simulink model "LKA_Lenkung_CarMaker_DSR_kombiniert_algSynth"  (Simulink 7.9)
settings: Solver=ode23  StartTime=0.0  StopTime=tend-1  FixedStep=0.01  RelTol=1e-3
undefined symbols (not defined in the file or in its folder): pin
libraries: library x5, simulink x3
settings Model: Creator=Georg  LastModifiedBy=georgnestlinger
settings DebuggingCC: FcnCallInpInsideContextMsg=Use local settings  StrictBusMsg=Warning
settings GRTTargetCC: CombineOutputUpdateFcns=off  GRTInterface=on

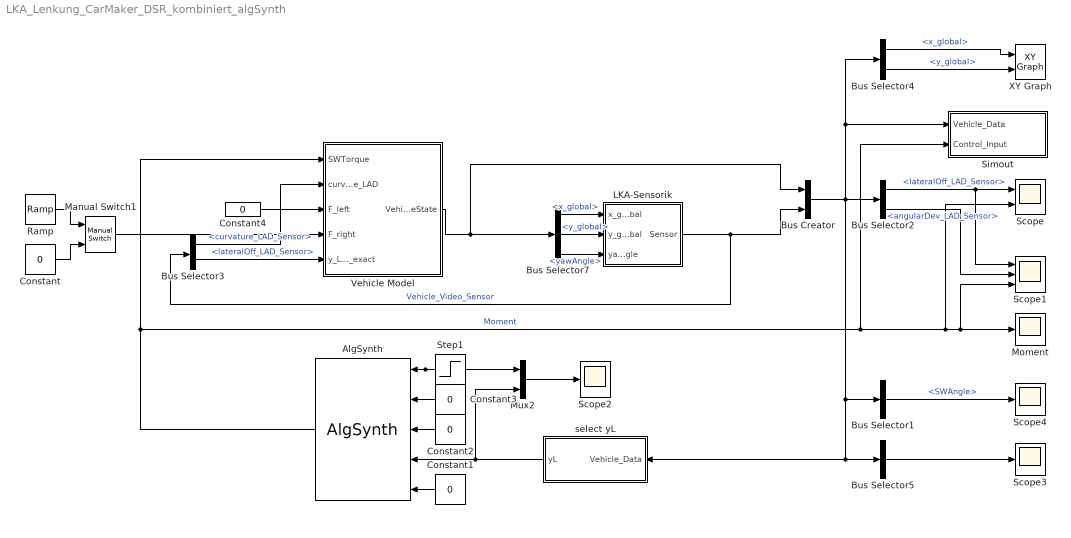
== system LKA_Lenkung_CarMaker_DSR_kombiniert_algSynth ==
  AlgSynth : library/LKA-Controller/AlgSynth
  Bus Creator : BusCreator  Inputs=2
  Bus Selector1 : BusSelector  OutputSignals=VehicleState.SWAngle
  Bus Selector2 : BusSelector  OutputSignals=Vehicle_Video_Sensor.lateralOff_LAD_Sensor,Vehicle_Video_Sensor.angularDev_LAD_Sensor
  Bus Selector3 : BusSelector  OutputSignals=curvature_LAD_Sensor,lateralOff_LAD_Sensor
  Bus Selector4 : BusSelector  OutputSignals=VehicleState.x_global,VehicleState.y_global
  Bus Selector5 : BusSelector  OutputSignals=VehicleState.angularDev_LAD_nonlinear,Vehicle_Video_Sensor.angularDev_LAD_Sensor  OutputAsBus=on
  Bus Selector7 : BusSelector  OutputSignals=x_global,y_global,yawAngle
  Constant{,1..4} (5 alike) : Constant  Value=0
  LKA-Sensorik : Subsystem  BlockChoice=Videosensorik
      settings: AttributesFormatString=%<BlockChoice>  TemplateBlock=library/LKA-Sensorik/LKA-Sensorik  MemberBlocks=Videosensorik
  Manual Switch1 : simulink/Signal Routing/Manual Switch  sw=0  action=0  varsize=off
  Moment : Scope
      settings: TimeRange=32.2  YMin=0.0002694  YMax=0.0002697  SaveName=ScopeData2
  Mux2 : Mux  Inputs=2
  Ramp : simulink/Sources/Ramp  slope=1  start=20  X0=0
  Scope : Scope  NumInputPorts=2
      settings: TimeRange=12.7664  YMin=-2.5e-06~-5e-05  YMax=3.25e-05~0.00025
  Scope1 : Scope  NumInputPorts=3
      settings: TimeRange=20  YMin=-5.5e-008~0.01711~-1.666e-008  YMax=5e-009~0.017145~-1.6565e-008
  Scope2 : Scope
      settings: TimeRange=5.66  YMin=0  YMax=1.05e-008  SaveName=ScopeData6
  Scope3 : Scope
      settings: YMin=0  YMax=0.035  SaveName=ScopeData3
  Scope4 : Scope
      settings: YMin=0.1675  YMax=0.205  SaveName=ScopeData4
  Simout : Subsystem
  Step1 : Step  Time=10  After=0  SampleTime=0
  Vehicle Model : Subsystem
  XY Graph : simulink/Sinks/XY Graph  xmin=-100  xmax=700  ymin=-1  ymax=600  st=-1
  select yL : Subsystem  BlockChoice=yL_Sensor
      settings: AttributesFormatString=%<BlockChoice>  TemplateBlock=library/LKA-Sensorik/select yL  MemberBlocks=yL_Sensor,yL_exactMdl,yL_linMdl
  wires:
  Bus Selector4/1 -> XY Graph/1  "<x_global>"
  Bus Selector4/2 -> XY Graph/2  "<y_global>"
  Bus Selector2/1 -> Scope/1, Scope1/1  "<lateralOff_LAD_Sensor>"
  Bus Selector2/2 -> Scope1/2  "<angularDev_LAD_Sensor>"
  Vehicle Model/1(VehicleState) -> Bus Creator/1, Bus Selector7/1
  LKA-Sensorik/1(Sensor) -> Bus Creator/2, Bus Selector3/1  "Vehicle_Video_Sensor"
  Bus Creator/1 -> Bus Selector2/1, Bus Selector1/1, Bus Selector5/1, select yL/1(Vehicle_Data), Bus Selector4/1, Simout/1(Vehicle_Data)
  Bus Selector5/1 -> Scope3/1
  Bus Selector1/1 -> Scope4/1  "<SWAngle>"
  Constant/1 -> Manual Switch1/2
  Manual Switch1/1 -> Vehicle Model/4(F_right)
  Bus Selector3/2 -> Vehicle Model/5(y_LAD_exact)  "<lateralOff_LAD_Sensor>"
  Bus Selector3/1 -> Vehicle Model/2(curvature_LAD)  "<curvature_LAD_Sensor>"
  select yL/1(yL) -> Mux2/2, AlgSynth/4
  AlgSynth/1 -> Scope/2, Scope1/3, Moment/1, Simout/2(Control_Input), Vehicle Model/1(SWTorque)  "Moment"
  Mux2/1 -> Scope2/1
  Step1/1 -> Mux2/1, AlgSynth/1
  Constant3/1 -> AlgSynth/2
  Constant2/1 -> AlgSynth/3
  Constant1/1 -> AlgSynth/5
  Constant4/1 -> Vehicle Model/3(F_left)
  Ramp/1 -> Manual Switch1/1
  Bus Selector7/1 -> LKA-Sensorik/1(x_global)  "<x_global>"
  Bus Selector7/2 -> LKA-Sensorik/2(y_global)  "<y_global>"
  Bus Selector7/3 -> LKA-Sensorik/3(yawAngle)  "<yawAngle>"

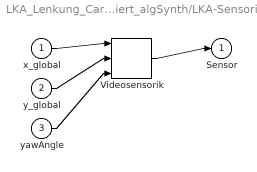
== system LKA_Lenkung_CarMaker_DSR_kombiniert_algSynth/LKA-Sensorik ==
  x_global : Inport
  y_global : Inport  Port=2
  yawAngle : Inport  Port=3
  Videosensorik : library/LKA-Sensorik/Videosensorik
  Sensor : Outport
  wires:
  x_global/1 -> Videosensorik/1
  y_global/1 -> Videosensorik/2
  yawAngle/1 -> Videosensorik/3
  Videosensorik/1 -> Sensor/1

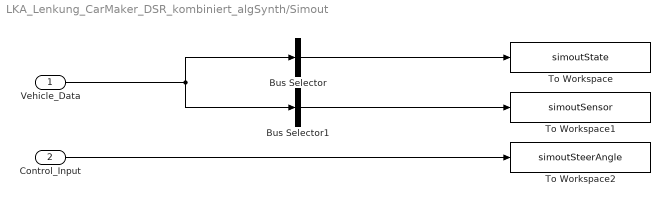
== system LKA_Lenkung_CarMaker_DSR_kombiniert_algSynth/Simout ==
  Vehicle_Data : Inport
  Control_Input : Inport  Port=2
  Bus Selector : BusSelector  OutputSignals=VehicleState  OutputAsBus=on
  Bus Selector1 : BusSelector  OutputSignals=Vehicle_Video_Sensor  OutputAsBus=on
  To Workspace : ToWorkspace  VariableName=simoutState  SampleTime=-1  SaveFormat=Structure With Time
  To Workspace1 : ToWorkspace  VariableName=simoutSensor  SampleTime=-1  SaveFormat=Structure With Time
  To Workspace2 : ToWorkspace  VariableName=simoutSteerAngle  SampleTime=-1  SaveFormat=Structure With Time
  wires:
  Vehicle_Data/1 -> Bus Selector1/1, Bus Selector/1
  Control_Input/1 -> To Workspace2/1
  Bus Selector/1 -> To Workspace/1
  Bus Selector1/1 -> To Workspace1/1

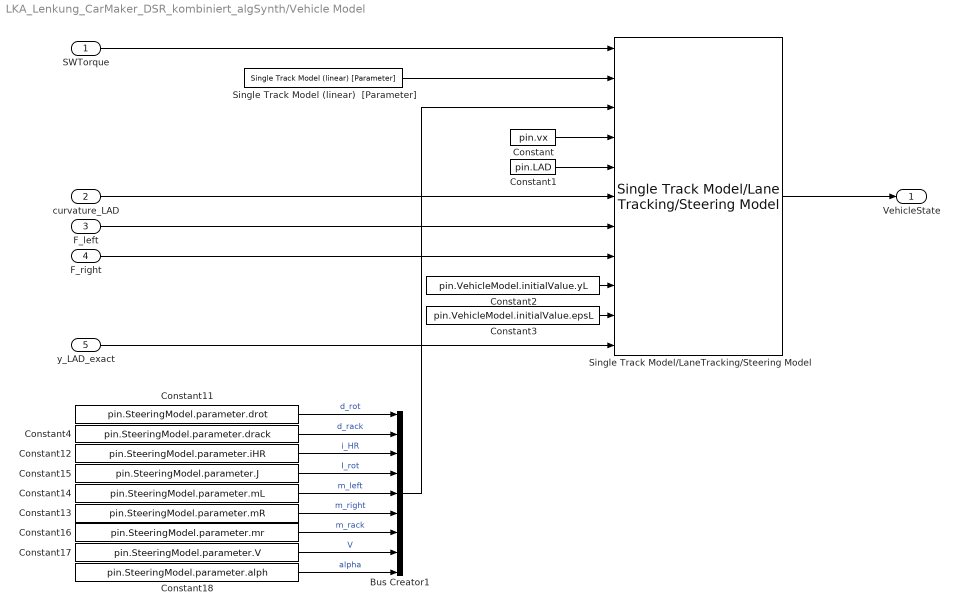
== system LKA_Lenkung_CarMaker_DSR_kombiniert_algSynth/Vehicle Model ==
  SWTorque : Inport
  curvature_LAD : Inport  Port=2
  F_left : Inport  Port=3
  F_right : Inport  Port=4
  y_LAD_exact : Inport  Port=5
  Bus Creator1 : BusCreator  Inputs=9
  Constant : Constant  Value=pin.vx
  Constant1 : Constant  Value=pin.LAD
  Constant11 : Constant  Value=pin.SteeringModel.parameter.drot
  Constant12 : Constant  Value=pin.SteeringModel.parameter.iHR
  Constant13 : Constant  Value=pin.SteeringModel.parameter.mR
  Constant14 : Constant  Value=pin.SteeringModel.parameter.mL
  Constant15 : Constant  Value=pin.SteeringModel.parameter.J
  Constant16 : Constant  Value=pin.SteeringModel.parameter.mr
  Constant17 : Constant  Value=pin.SteeringModel.parameter.V
  Constant18 : Constant  Value=pin.SteeringModel.parameter.alph
  Constant2 : Constant  Value=pin.VehicleModel.initialValue.yL
  Constant3 : Constant  Value=pin.VehicleModel.initialValue.epsL
  Constant4 : Constant  Value=pin.SteeringModel.parameter.drack
  Single Track Model (linear)  [Parameter] : library/Vehicle Models/Single Track Models/Single Track Model (linear) [Parameter]  cs_front=pin.VehicleModel.parameter.csv  cs_rear=pin.VehicleModel.parameter.csh  l_front=pin.VehicleModel.parameter.lv  l_rear=pin.VehicleModel.parameter.lh  m=pin.VehicleModel.parameter.m  Izz=pin.VehicleModel.parameter.Iz
  Single Track Model/LaneTracking/Steering Model : library/Vehicle Models/Single Track Model//Lane Tracking//Steering Model
  VehicleState : Outport
  wires:
  curvature_LAD/1 -> Single Track Model/LaneTracking/Steering Model/6
  Bus Creator1/1 -> Single Track Model/LaneTracking/Steering Model/3
  Constant/1 -> Single Track Model/LaneTracking/Steering Model/4
  Constant1/1 -> Single Track Model/LaneTracking/Steering Model/5
  Single Track Model/LaneTracking/Steering Model/1 -> VehicleState/1
  F_left/1 -> Single Track Model/LaneTracking/Steering Model/7
  F_right/1 -> Single Track Model/LaneTracking/Steering Model/8
  Constant2/1 -> Single Track Model/LaneTracking/Steering Model/9
  Constant3/1 -> Single Track Model/LaneTracking/Steering Model/10
  y_LAD_exact/1 -> Single Track Model/LaneTracking/Steering Model/11
  SWTorque/1 -> Single Track Model/LaneTracking/Steering Model/1
  Single Track Model (linear)  [Parameter]/1 -> Single Track Model/LaneTracking/Steering Model/2
  Constant11/1 -> Bus Creator1/1  "d_rot"
  Constant4/1 -> Bus Creator1/2  "d_rack"
  Constant12/1 -> Bus Creator1/3  "i_HR"
  Constant15/1 -> Bus Creator1/4  "I_rot"
  Constant14/1 -> Bus Creator1/5  "m_left"
  Constant13/1 -> Bus Creator1/6  "m_right"
  Constant16/1 -> Bus Creator1/7  "m_rack"
  Constant17/1 -> Bus Creator1/8  "V"
  Constant18/1 -> Bus Creator1/9  "alpha"

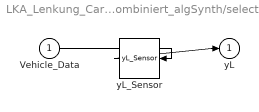
== system LKA_Lenkung_CarMaker_DSR_kombiniert_algSynth/select yL ==
  Vehicle_Data : Inport
  yL_Sensor : library/LKA-Sensorik/yL_Sensor
  yL : Outport
  wires:
  Vehicle_Data/1 -> yL_Sensor/1
  yL_Sensor/1 -> yL/1
